simulink model "draft4_2014b"  (R2014b)
settings: Solver=FixedStepDiscrete  SolverMode=SingleTasking  StartTime=0.0  StopTime=10.0  RelTol=1e-3
settings Model: CovMetricSettings=dwe  CovHtmlReporting=off  covSaveCumulativeToWorkspaceVar=off  CovSaveSingleToWorkspaceVar=off  CovExternalEMLEnable=on  CovSFcnEnable=on  Creator=hbourbou  LastModifiedBy=hbourbou
settings DataIOCC: LimitDataPoints=off  SaveFormat=StructureWithTime
settings DebuggingCC: SolverPrmCheckMsg=none  FrameProcessingCompatibilityMsg=error  SFUnexpectedBacktrackingDiag=error  SFNoUnconditionalDefaultTransitionDiag=error
settings HardwareCC: ProdBitPerPointer=64  ProdLargestAtomicFloat=Float  ProdIntDivRoundTo=Zero  ProdEndianess=LittleEndian  ProdHWDeviceType=Specified
settings ModelReferenceCC: PropagateSignalLabelsOutOfModel=on
settings GRTTargetCC: TargetLangStandard=C99 (ISO)  GeneratePreprocessorConditionals=Use local settings

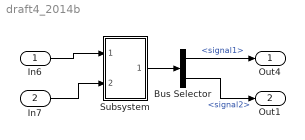
== system draft4_2014b ==
  In6 : Inport  OutDataTypeStr=double
  In7 : Inport  Port=2  OutDataTypeStr=boolean
  Bus Selector : BusSelector  OutputSignals=signal1,signal2
  Subsystem : Subsystem  TreatAsAtomicUnit=on
  Out4 : Outport
  Out1 : Outport  Port=2
  wires:
  Bus Selector/1 -> Out4/1  "<signal1>"
  Bus Selector/2 -> Out1/1  "<signal2>"
  In6/1 -> Subsystem/1(In6)
  In7/1 -> Subsystem/2(In7)
  Subsystem/1(Out1) -> Bus Selector/1

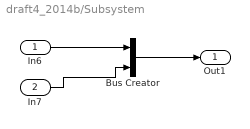
== system draft4_2014b/Subsystem ==
  In6 : Inport  OutDataTypeStr=double
  In7 : Inport  Port=2  OutDataTypeStr=boolean
  Bus Creator : BusCreator  Inputs=2  OutDataTypeStr=Bus: db
  Out1 : Outport
  wires:
  In7/1 -> Bus Creator/2
  Bus Creator/1 -> Out1/1
  In6/1 -> Bus Creator/1
